simulink model "Problem3"  (R2020b)
settings: Solver=VariableStepAuto  StartTime=0.0  StopTime=0.1  RelTol=1e-3
settings Model: Creator=hp  LastModifiedBy=hp

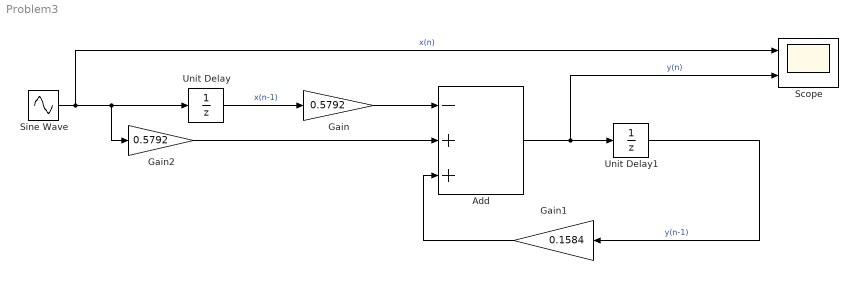
== system Problem3 ==
  Add : Sum  Inputs=-++
  Gain : Gain  Gain=0.5792
  Gain1 : Gain  Gain=0.1584
  Gain2 : Gain  Gain=0.5792
  Scope : Scope  NumInputPorts=2
  Sine Wave : Sin  Frequency=2*pi*760  SampleTime=1/5000
  Unit Delay : UnitDelay  SampleTime=-1  HasFrameUpgradeWarning=on
  Unit Delay1 : UnitDelay  SampleTime=-1  HasFrameUpgradeWarning=on
  wires:
  Sine Wave/1 -> Scope/1, Gain2/1, Unit Delay/1  "x(n)"
  Unit Delay/1 -> Gain/1  "x(n-1)"
  Gain/1 -> Add/1
  Add/1 -> Scope/2, Unit Delay1/1  "y(n)"
  Unit Delay1/1 -> Gain1/1  "y(n-1)"
  Gain1/1 -> Add/3
  Gain2/1 -> Add/2
